simulink model "Controlador_Cascada_RMS_obs_a_mano"  (R2020a)
settings: Solver=ode15s  StartTime=0.0  StopTime=10.0  MaxStep=0.0001  RelTol=1e-3
undefined symbols (not defined in the file): Amp, Aobs, ba, bm, Bobs, C_obs, f, K_motor, K_motor_virtual, k_resorte, Kcorr, Ki, ksi, ksia, Kv, Kx, L, Lobs, m_total, R, R_control
libraries: dspstat3 x1
settings Model: Creator=Adriana  LastModifiedBy=Noxi-PC

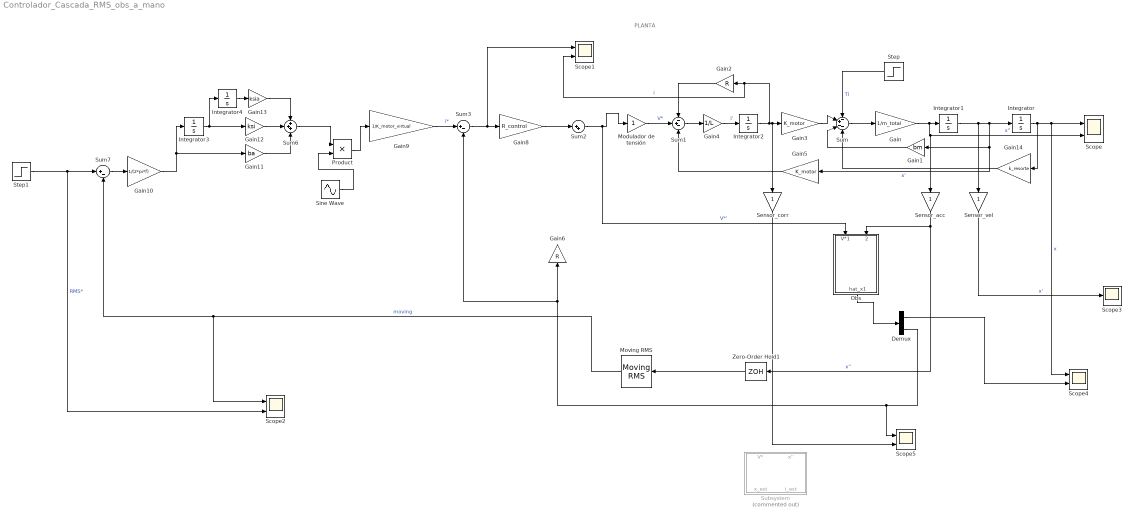
== system Controlador_Cascada_RMS_obs_a_mano ==
  note: PLANTA
  " Sensor_acc" : Gain
  " Sensor_vel" : Gain
  Demux : Demux  Outputs=3
  Gain : Gain  Gain=1/m_total
  Gain1 : Gain  Gain=bm
  Gain10 : Gain  Gain=1/(2*pi*f)
  Gain11 : Gain  Gain=ba
  Gain12 : Gain  Gain=ksi
  Gain13 : Gain  Gain=ksia
  Gain14 : Gain  Gain=k_resorte
  Gain2 : Gain  Gain=R
  Gain3 : Gain  Gain=K_motor
  Gain4 : Gain  Gain=1/L
  Gain5 : Gain  Gain=K_motor
  Gain6 : Gain  Gain=R
  Gain8 : Gain  Gain=R_control
  Gain9 : Gain  Gain=1/K_motor_virtual
  Integrator{,1..4} (5 alike) : Integrator
  Modulador de tensión : Gain
  Moving RMS : dspstat3/Moving RMS  Method=Sliding window  ForgettingFactorPort=off  SpecifyWindowLength=on  WindowLength=Ventana  ForgettingFactor=0.99  SimulateUsing=Code generation
      settings: SourceProductBaseCode=DS
  Obs : Subsystem
  Product : Product
  Scope{,1..2,4..5} (5 alike) : Scope  NumInputPorts=2
  Scope3 : Scope
  Sensor_corr : Gain
  Sine Wave : Sin  Frequency=2*pi*f  SampleTime=0
  Step : Step  Time=3  After=0  SampleTime=0
  Step1 : Step  After=Amp/sqrt(2)  SampleTime=0
  Subsystem : Subsystem  Commented=on
  Sum : Sum  Inputs=-+--
  Sum1 : Sum  Inputs=-+-
  Sum2 : Sum  Inputs=|++
  Sum3 : Sum  Inputs=|+-
  Sum6 : Sum  Inputs=+++
  Sum7 : Sum  Inputs=|+-
  Zero-Order Hold1 : ZeroOrderHold  SampleTime=0.001
  wires:
  Integrator1/1 -> " Sensor_vel"/1, Gain5/1, Gain1/1, Integrator/1  "x'"
  Integrator/1 -> Gain14/1, Scope4/1, Scope/1  "x"
  Gain/1 -> Scope/2, " Sensor_acc"/1, Integrator1/1  "x''"
  Sum/1 -> Gain/1
  Gain1/1 -> Sum/3
  Step/1 -> Sum/1  "Tl"
  Gain3/1 -> Sum/2
  Integrator2/1 -> Scope1/2, Gain2/1, Gain3/1, Sensor_corr/1  "i"
  Sum1/1 -> Gain4/1
  Gain4/1 -> Integrator2/1  "i'"
  Gain2/1 -> Sum1/1
  Gain5/1 -> Sum1/3
  Modulador de tensión/1 -> Sum1/2  "V*"
  Sum2/1 -> Obs/1(V*1), Modulador de tensión/1  "V*'"
  " Sensor_vel"/1 -> Scope3/1  "x'"
  Gain8/1 -> Sum2/1
  Sum3/1 -> Scope1/1, Gain8/1
  Gain9/1 -> Sum3/1  "i*"
  Integrator4/1 -> Gain13/1
  Integrator3/1 -> Integrator4/1, Gain12/1
  Gain12/1 -> Sum6/2
  Gain13/1 -> Sum6/1
  Sum7/1 -> Gain10/1
  Gain11/1 -> Sum6/3
  Gain14/1 -> Sum/4
  Moving RMS/1 -> Scope2/1, Sum7/2  "moving"
  Zero-Order Hold1/1 -> Moving RMS/1
  Step1/1 -> Scope2/2, Sum7/1  "RMS*"
  Gain10/1 -> Integrator3/1, Gain11/1
  Sum6/1 -> Product/1
  Product/1 -> Gain9/1
  Sine Wave/1 -> Product/2
  Obs/1(hat_x1) -> Demux/1
  " Sensor_acc"/1 -> Obs/2(acc_medida1), Zero-Order Hold1/1  "x''"
  Demux/3 -> Scope5/1, Sum3/2, Gain6/1
  Demux/1 -> Scope4/2
  Sensor_corr/1 -> Scope5/2

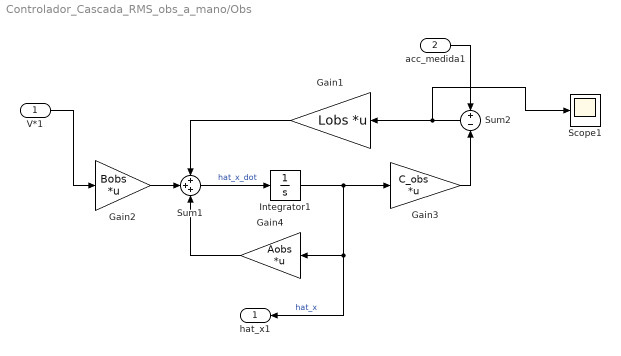
== system Controlador_Cascada_RMS_obs_a_mano/Obs ==
  V*1 : Inport
  acc_medida1 : Inport  Port=2
  Gain1 : Gain  Gain=Lobs  Multiplication=Matrix(K*u)
  Gain2 : Gain  Gain=Bobs  Multiplication=Matrix(K*u)
  Gain3 : Gain  Gain=C_obs  Multiplication=Matrix(K*u)
  Gain4 : Gain  Gain=Aobs  Multiplication=Matrix(K*u)
  Integrator1 : Integrator
  Scope1 : Scope
  Sum1 : Sum  Inputs=+++
  Sum2 : Sum  Inputs=+|-
  hat_x1 : Outport  VectorParamsAs1DForOutWhenUnconnected=off
  wires:
  Gain1/1 -> Sum1/1
  Gain4/1 -> Sum1/3
  V*1/1 -> Gain2/1
  Gain2/1 -> Sum1/2
  Sum2/1 -> Scope1/1, Gain1/1
  Integrator1/1 -> hat_x1/1, Gain4/1, Gain3/1  "hat_x"
  Sum1/1 -> Integrator1/1  "hat_x_dot"
  acc_medida1/1 -> Sum2/1
  Gain3/1 -> Sum2/2

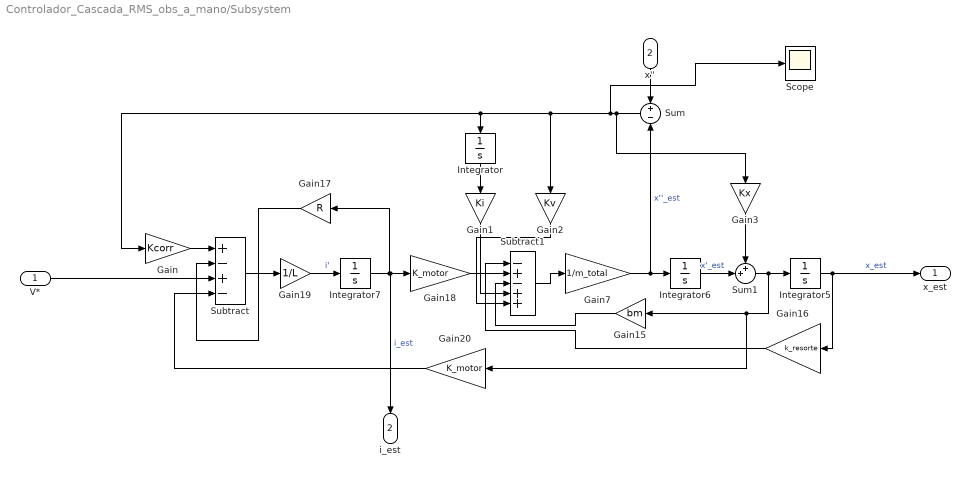
== system Controlador_Cascada_RMS_obs_a_mano/Subsystem ==
  V* : Inport
  x'' : Inport  Port=2
  Gain : Gain  Gain=Kcorr
  Gain1 : Gain  Gain=Ki
  Gain15 : Gain  Gain=bm
  Gain16 : Gain  Gain=k_resorte
  Gain17 : Gain  Gain=R
  Gain18 : Gain  Gain=K_motor
  Gain19 : Gain  Gain=1/L
  Gain2 : Gain  Gain=Kv
  Gain20 : Gain  Gain=K_motor
  Gain3 : Gain  Gain=Kx
  Gain7 : Gain  Gain=1/m_total
  Integrator{,5..7} (4 alike) : Integrator
  Scope : Scope
  Subtract : Sum  Inputs=+-+-
  Subtract1 : Sum  Inputs=-+-++
  Sum : Sum  Inputs=+-
  Sum1 : Sum  Inputs=++|
  x_est : Outport
  i_est : Outport  Port=2
  wires:
  Integrator7/1 -> i_est/1, Gain18/1, Gain17/1  "i_est"
  Subtract/1 -> Gain19/1
  Gain7/1 -> Sum/2, Integrator6/1  "x''_est"
  Gain15/1 -> Subtract1/3
  Gain16/1 -> Subtract1/1
  Gain17/1 -> Subtract/2
  Integrator5/1 -> x_est/1, Gain16/1  "x_est"
  Gain18/1 -> Subtract1/2
  Gain20/1 -> Subtract/4
  Gain19/1 -> Integrator7/1  "i'"
  V*/1 -> Subtract/3
  x''/1 -> Sum/1
  Gain/1 -> Subtract/1
  Sum/1 -> Scope/1, Gain2/1, Gain/1, Integrator/1, Gain3/1
  Subtract1/1 -> Gain7/1
  Gain1/1 -> Subtract1/4
  Gain2/1 -> Subtract1/5
  Integrator/1 -> Gain1/1
  Sum1/1 -> Gain20/1, Gain15/1, Integrator5/1
  Integrator6/1 -> Sum1/2  "x'_est"
  Gain3/1 -> Sum1/1
